simulink model "BlockDrag"  (R2020b)
settings: Solver=VariableStepAuto  StartTime=0.0  StopTime=tf  MaxStep=maxstep  RelTol=tol  AbsTol=tol
values from neighbouring files (symbols this model uses):
  b = 1    [BlockDragM.m]
  F = 10    [BlockDragM.m]    (also in Schimmel_Evan_lab_1_script.m = 6)
  m = 1    [BlockDragM.m]    (also in Schimmel_Evan_lab_1_script.m = 2)
  v0 = 1    [BlockDragM.m]    (also in Schimmel_Evan_lab_1_script.m = -1)
settings Model: Creator=schimmer  LastModifiedBy=schimmer
settings DataIOCC: SaveOutput=off  SignalLogging=off  DSMLogging=off  SaveTime=off  ReturnWorkspaceOutputs=off

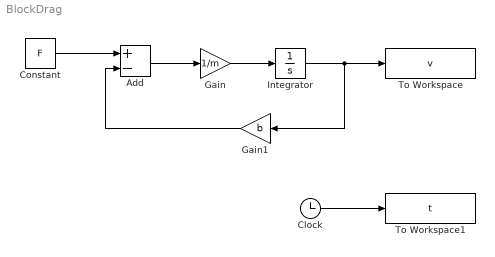
== system BlockDrag ==
  Add : Sum  Inputs=+-
  Clock : Clock
  Constant : Constant  Value=F
  Gain : Gain  Gain=1/m
  Gain1 : Gain  Gain=b
  Integrator : Integrator  InitialCondition=v0
  To Workspace : ToWorkspace  VariableName=v  SampleTime=-1
  To Workspace1 : ToWorkspace  VariableName=t  SampleTime=-1
  wires:
  Gain/1 -> Integrator/1
  Integrator/1 -> Gain1/1, To Workspace/1
  Add/1 -> Gain/1
  Gain1/1 -> Add/2
  Constant/1 -> Add/1
  Clock/1 -> To Workspace1/1
